simulink model "example_EU_Tapping"  (R2018b)
settings: Solver=ode45  StartTime=0.0  StopTime=24*3600  MaxStep=60  RelTol=1e-3  EnableMultiTasking=on
libraries: carnot x7
settings Model: Creator=drhf  LastModifiedBy=drhf
settings DataIOCC: LimitDataPoints=on  SaveFormat=Array
settings OptimizationCC: ExpressionDepthLimit=2147483647  LifeSpan=inf
settings DebuggingCC: UnderspecifiedInitializationDetection=Classic  MergeDetectMultiDrivingBlocksExec=none  SolverPrmCheckMsg=warning  StateNameClashWarn=warning  SFUnexpectedBacktrackingDiag=warning  SFNoUnconditionalDefaultTransitionDiag=warning  SFExecutionAtInitializationDiag=none
settings HardwareCC: ProdBitPerPointer=32  ProdBitPerSizeT=32  ProdBitPerPtrDiffT=32  ProdLargestAtomicFloat=None  ProdIntDivRoundTo=Undefined  ProdEndianess=Unspecified  ProdWordSize=32  ProdHWDeviceType=32-bit Generic
settings ModelReferenceCC: PropagateSignalLabelsOutOfModel=off
settings SFSimCC: SimUseLocalCustomCode=off
settings RTWCC: RTWUseLocalCustomCode=off
settings CodeAppCC: StateflowObjectComments=on
settings GRTTargetCC: TargetLangStandard=C89/C90 (ANSI)  GeneratePreprocessorConditionals=Disable all  CombineOutputUpdateFcns=off  GRTInterface=on
settings ConfigComp: CovMetricSettings=dw  CovHtmlReporting=on  CovSaveCumulativeToWorkspaceVar=on  CovSaveSingleToWorkspaceVar=on  CovExternalEMLEnable=off

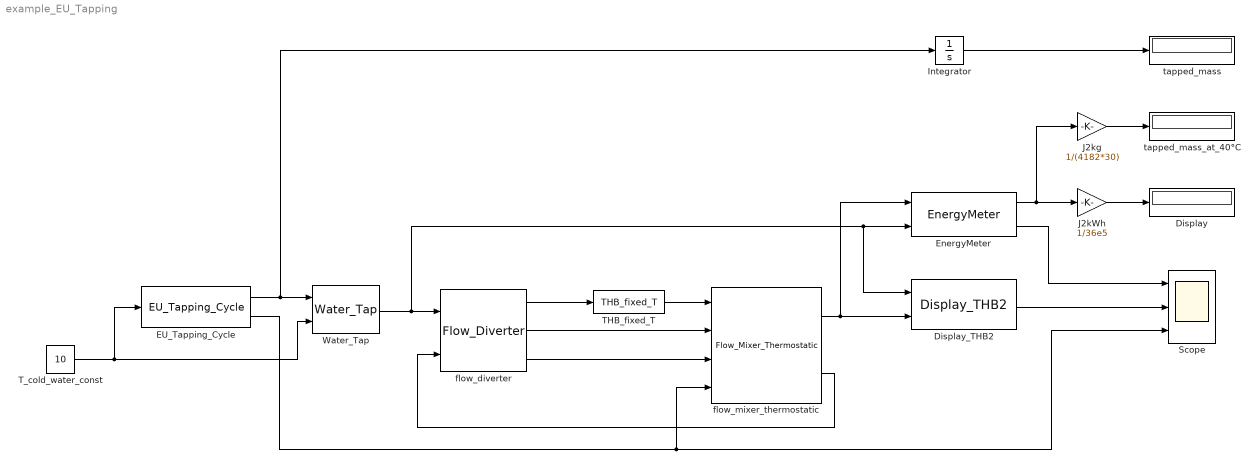
== system example_EU_Tapping ==
  Display : Display
  Display_THB2 : carnot/Outputs/Display_THB2  t=off  m=on  p=off  id=off  mix=off  d=off
      settings: SourceProductName=Carnot
  EU_Tapping_Cycle : carnot/Load/Hot_Water_Tapping/EU_Tapping_Cycle  eu_tap=M  dTbias=0
      settings: SourceProductName=Carnot
  EnergyMeter : carnot/Control/EnergyMeter
      settings: SourceProductName=Carnot
  Integrator : Integrator
  J2kWh : Gain  Gain=1/36e5
  J2kg : Gain  Gain=1/(4182*30)
  Scope : Scope  NumInputPorts=3
  THB_fixed_T : carnot/Source/Simple/THB_fixed_T  t=60
      settings: SourceProductName=Carnot
  T_cold_water_const : Constant  Value=10
  Water_Tap : carnot/Load/Hot_Water_Tapping/Water_Tap  dia=0.02  p=2e5
      settings: SourceProductName=Carnot
  flow_diverter : carnot/Hydraulics/Flow_Diverter
      settings: SourceProductName=Carnot
  flow_mixer_thermostatic : carnot/Hydraulics/Flow_Mixer_Thermostatic  t=10
      settings: SourceProductName=Carnot
  tapped_mass : Display
  tapped_mass_at_40°C : Display
  wires:
  Display_THB2/1 -> Scope/2
  EnergyMeter/1 -> J2kg/1, J2kWh/1
  J2kWh/1 -> Display/1
  EnergyMeter/2 -> Scope/1
  Water_Tap/1 -> flow_diverter/1, Display_THB2/1, EnergyMeter/2
  T_cold_water_const/1 -> Water_Tap/2, EU_Tapping_Cycle/1
  EU_Tapping_Cycle/1 -> Integrator/1, Water_Tap/1
  flow_diverter/3 -> flow_mixer_thermostatic/3
  flow_diverter/2 -> flow_mixer_thermostatic/2
  THB_fixed_T/1 -> flow_mixer_thermostatic/1
  flow_mixer_thermostatic/1 -> Display_THB2/2, EnergyMeter/1
  flow_mixer_thermostatic/2 -> flow_diverter/2
  flow_diverter/1 -> THB_fixed_T/1
  Integrator/1 -> tapped_mass/1
  J2kg/1 -> tapped_mass_at_40°C/1
  EU_Tapping_Cycle/2 -> Scope/3, flow_mixer_thermostatic/4
